simulink model "SICOsimulink_model"  (R2017b)
settings: Solver=VariableStepAuto  StartTime=0.0  StopTime=57  RelTol=1e-3
settings Model: Creator=ladislav  LastModifiedBy=ladislav

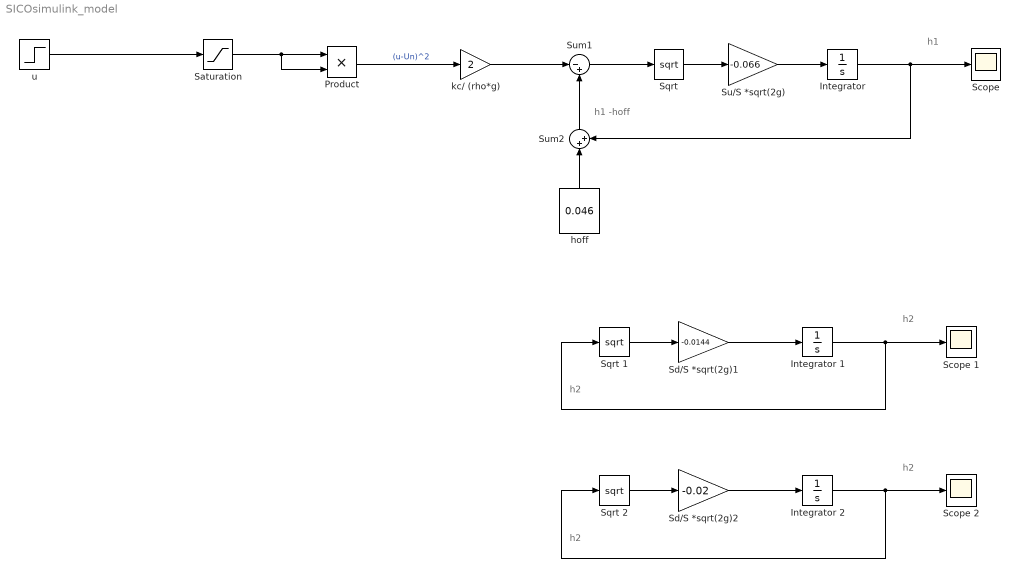
== system SICOsimulink_model ==
  note: h1
  note: h1 -hoff
  note: h2
  note: h2
  note: h2
  note: h2
  " hoff" : Constant  Value=0.046
  "Integrator " : Integrator  InitialCondition=0.1582
  Integrator 1 : Integrator  InitialCondition=0.14
  Integrator 2 : Integrator  InitialCondition=0.146
  "Product " : Product
  "Saturation " : Saturate  UpperLimit=1  LowerLimit=0.05
  "Scope " : Scope
  Scope 1 : Scope
  Scope 2 : Scope
  Sd/S *sqrt(2g)1 : Gain  Gain=-0.0144
  Sd/S *sqrt(2g)2 : Gain  Gain=-0.02
  "Sqrt " : Sqrt  SaturateOnIntegerOverflow=on
  Sqrt 1 : Sqrt  SaturateOnIntegerOverflow=on
  Sqrt 2 : Sqrt  SaturateOnIntegerOverflow=on
  Su/S *sqrt(2g) : Gain  Gain=-0.066
  Sum1 : Sum  Inputs=|-+
  Sum2 : Sum  Inputs=|++
  kc/ (rho*g) : Gain  Gain=2
  u : Step  After=0  SampleTime=0
  wires:
  u/1 -> "Saturation "/1
  "Saturation "/1 -> "Product "/2, "Product "/1
  "Product "/1 -> kc/ (rho*g)/1  "(u-Un)^2"
  Sum1/1 -> "Sqrt "/1
  "Sqrt "/1 -> Su/S *sqrt(2g)/1
  Su/S *sqrt(2g)/1 -> "Integrator "/1
  Sum2/1 -> Sum1/2
  " hoff"/1 -> Sum2/1
  "Integrator "/1 -> "Scope "/1, Sum2/2
  Sd/S *sqrt(2g)1/1 -> Integrator 1/1
  Integrator 1/1 -> Sqrt 1/1, Scope 1/1
  Sqrt 1/1 -> Sd/S *sqrt(2g)1/1
  kc/ (rho*g)/1 -> Sum1/1
  Integrator 2/1 -> Sqrt 2/1, Scope 2/1
  Sd/S *sqrt(2g)2/1 -> Integrator 2/1
  Sqrt 2/1 -> Sd/S *sqrt(2g)2/1
